simulink model "ECC_Chain"  (R2025b)
settings: Solver=VariableStepAuto  StartTime=0.0  StopTime=10.0  RelTol=1e-3
settings Model: Creator=strog  LastModifiedBy=strog

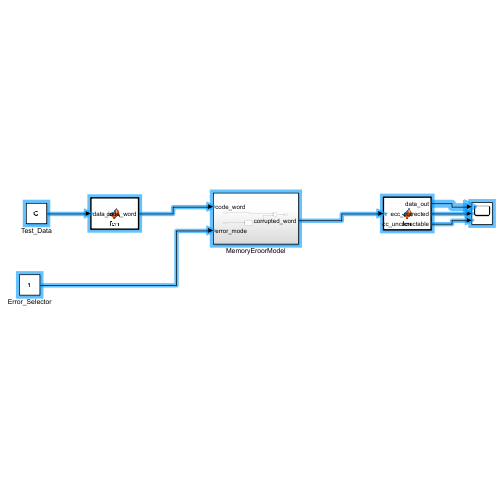
[thumbnail: Simulink's stored preview of the top-level diagram]
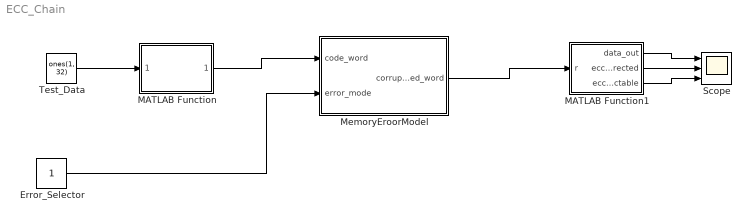
== system ECC_Chain ==
  Error_Selector : Constant  OutDataTypeStr=boolean
  MATLAB Function : MATLAB Function  TreatAsAtomicUnit=on
  MATLAB Function1 : MATLAB Function  TreatAsAtomicUnit=on
  MemoryEroorModel : Subsystem
  Scope : Scope  NumInputPorts=3
      settings: DataLoggingSaveFormat=Array
  Test_Data : Constant  Value=ones(1, 32)  OutDataTypeStr=boolean
  wires:
  MATLAB Function1/3(ecc_uncorrectable) -> Scope/3
  MATLAB Function1/2(ecc_corrected) -> Scope/2
  MATLAB Function/1(code_word) -> MemoryEroorModel/1(code_word)
  Error_Selector/1 -> MemoryEroorModel/2(error_mode)
  MemoryEroorModel/1(corrupted_word) -> MATLAB Function1/1(r)
  Test_Data/1 -> MATLAB Function/1(data_in)
  MATLAB Function1/1(data_out) -> Scope/1

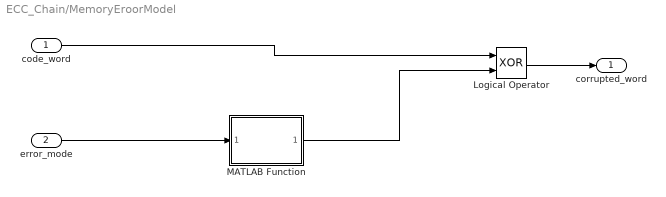
== system ECC_Chain/MemoryEroorModel ==
  code_word : Inport
  error_mode : Inport  Port=2
  Logical Operator : Logic  Operator=XOR  AllPortsSameDT=off  OutDataTypeStr=boolean
  MATLAB Function : MATLAB Function  TreatAsAtomicUnit=on
  corrupted_word : Outport
  wires:
  code_word/1 -> Logical Operator/1
  error_mode/1 -> MATLAB Function/1(error_mode)
  MATLAB Function/1(error_mask) -> Logical Operator/2
  Logical Operator/1 -> corrupted_word/1

== matlab function ECC_Chain/MATLAB Function ==
  data: data_in input; code_word output
function code_word = fcn(data_in)
    % data_in: вектор из 32 элементов (uint8 или логический), содержащий биты данных
    % code_word: выходной вектор из 39 бит
    
    % Инициализируем кодовое слово нулями
    c = zeros(1, 39);
    
    % Размещаем 32 бита информационных данных на позиции, не являющиеся степенями двойки
    % Позиции контрольных бит: 1, 2, 4, 8, 16, 32
    % Позиция 39 — общий бит четности (для превращения SEC в SECDED)
    
    data_pos =;
    
    for i = 1:32
        c(data_pos(i)) = data_in(i);
    end
    
    % Вычисляем контрольные биты Хэмминга (XOR по соответствующим позициям)
    c(1)  = mod(sum(c([3, 5, 7, 9, 11, 13, 15, 17, 19, 21, 23, 25, 27, 29, 31, 33, 35, 37])), 2);
    c(2)  = mod(sum(c([3, 6, 7, 10, 11, 14, 15, 18, 19, 22, 23, 26, 27, 30, 31, 34, 35, 38])), 2);
    c(4)  = mod(sum(c([5, 6, 7, 12, 13, 14, 15, 20, 21, 22, 23, 28, 29, 30, 31, 36, 37, 38])), 2);
    c(8)  = mod(sum(c([9:15, 24:31, 38])), 2); % для сокращенного кода проверяем доступные диапазоны
    c(16) = mod(sum(c([17:31])), 2);
    c(32) = mod(sum(c([33:38])), 2);
    
    % 39-й бит: Общий паритет (SECDED) — XOR всех предыдущих 38 бит
    c(39) = mod(sum(c(1:38)), 2);
    
    code_word = c;
end

== matlab function ECC_Chain/MemoryEroorModel/MATLAB Function ==
  data: error_mode input; error_mask output
function error_mask = fcn(error_mode)
    % error_mode: 0, 1 или 2
    % error_mask: вектор из 39 бит (0 или 1)
    
    error_mask = zeros(1, 39);
    
    if error_mode == 1
        % Вносим ровно 1 ошибку в фиксированную (например, 5-ю) позицию
        error_mask(5) = 1; 
    elseif error_mode == 2
        % Вносим ровно 2 ошибки (например, в 5-ю и 12-ю позиции)
        error_mask(5) = 1;
        error_mask(12) = 1;
    end
end

== matlab function ECC_Chain/MATLAB Function1 ==
  data: r input; data_out output; ecc_corrected output; ecc_uncorrectable output
function [data_out, ecc_corrected, ecc_uncorrectable] = fcn(r)
    % r: принятое из памяти 39-битное слово
    
    % Инициализация флагов
    ecc_corrected = 0;
    ecc_uncorrectable = 0;
    
    % 1. Вычисляем синдром Хэмминга (6 бит)
    s = zeros(1, 6);
    s(1) = mod(sum(r([1, 3, 5, 7, 9, 11, 13, 15, 17, 19, 21, 23, 25, 27, 29, 31, 33, 35, 37])), 2);
    s(2) = mod(sum(r([2, 3, 6, 7, 10, 11, 14, 15, 18, 19, 22, 23, 26, 27, 30, 31, 34, 35, 38])), 2);
    s(3) = mod(sum(r([4, 5, 6, 7, 12, 13, 14, 15, 20, 21, 22, 23, 28, 29, 30, 31, 36, 37, 38])), 2);
    s(4) = mod(sum(r([8:15, 24:31, 38])), 2);
    s(5) = mod(sum(r([16:31])), 2);
    s(6) = mod(sum(r([32:38])), 2);
    
    % Преобразуем синдром в десятичное число (индекс ошибочного бита)
    syndrome_val = s(1)*1 + s(2)*2 + s(3)*4 + s(4)*8 + s(5)*16 + s(6)*32;
    
    % 2. Вычисляем общий паритет принятого слова
    overall_parity = mod(sum(r), 2); % Если ошибок нет, общий паритет должен быть равен 0
    
    % 3. Логика SECDED декодирования
    if syndrome_val == 0
        if overall_parity == 0
            % Ошибок нет
        else
            % Ошибка в самом бите общего паритета (39)
            r(39) = mod(r(39) + 1, 2);
            ecc_corrected = 1;
        end
    else
        if overall_parity == 1
            % Одиночная ошибка (SEC) — исправляем её
            if syndrome_val <= 39
                r(syndrome_val) = mod(r(syndrome_val) + 1, 2);
                ecc_corrected = 1;
            end
        else
            % Двойная ошибка (DED) — обнаружена, но неисправима
            ecc_uncorrectable = 1;
        end
    end
    
    % Извлекаем чистые 32 бита данных из исправленного слова
    data_pos =;
    data_out = zeros(1, 32);
    for i = 1:32
        data_out(i) = r(data_pos(i));
    end
end
